simulink model "BLDC_FOC_Universal_Controller"  (R2025b)
settings: Solver=ode4  StartTime=0.0  StopTime=2  FixedStep=1e-5  RelTol=1e-3
undefined symbols (not defined in the file or in its folder): CurrentMotor_Imax, CurrentMotor_J, CurrentMotor_Kt, CurrentMotor_L, CurrentMotor_P, CurrentMotor_R, CurrentMotor_SpeedRef
libraries: fl_lib x13, nesl_utility x10, slpidlib x3, mcbeeMathTransformLib x2, eeTransforms x2, ee_lib x1
settings Model: Creator=metro  LastModifiedBy=metro

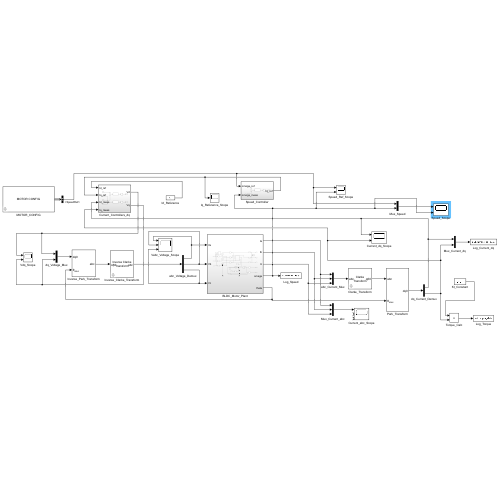
[thumbnail: Simulink's stored preview of the top-level diagram]
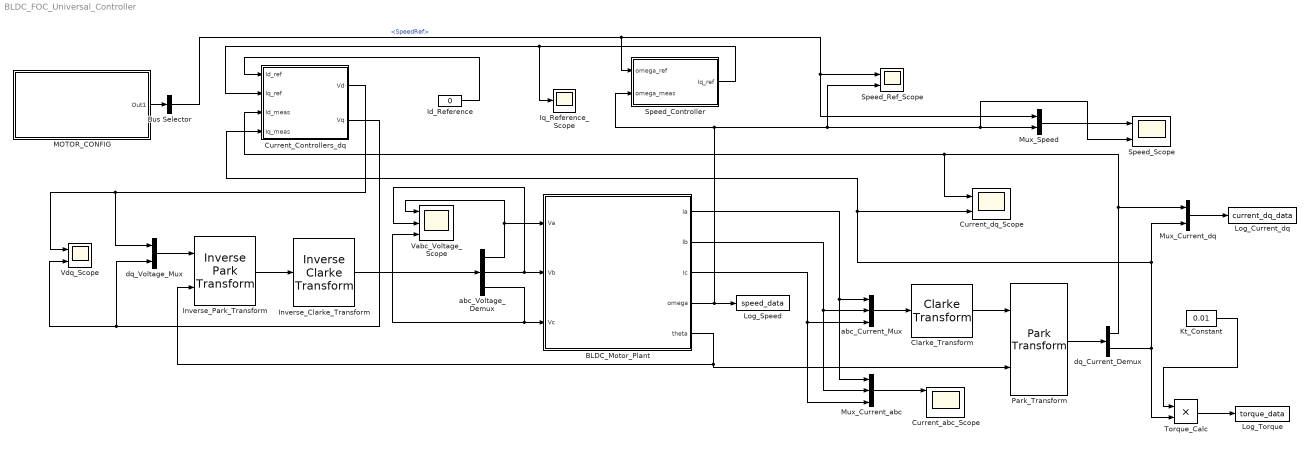
== system BLDC_FOC_Universal_Controller ==
  BLDC_Motor_Plant : Subsystem
  Bus Selector : BusSelector  OutputSignals=SpeedRef
  Clarke_Transform : mcbeeMathTransformLib/Clarke Transform  PowerInvariant=off  UseWithEmbedded=off  PhaseInput=Two inputs
      settings: LibrarySourceBlock=|
      | ee_sl_lib/Mathematical
      | Transforms/Clarke Transform
  Current_Controllers_dq : Subsystem
  Current_abc_Scope : Scope  NumInputPorts=3
      settings: ActiveDisplayYMinimum=-7.7006868638074586  ActiveDisplayYMaximum=10.228611642357857
  Current_dq_Scope : Scope  NumInputPorts=2
      settings: ActiveDisplayYMinimum=-9.97101009316468  ActiveDisplayYMaximum=4.854374604366809
  Id_Reference : Constant  Value=0
  Inverse_Clarke_Transform : mcbeeMathTransformLib/Inverse Clarke Transform  PowerInvariant=off  UseWithEmbedded=off  PhaseInput=Two inputs
      settings: LibrarySourceBlock=|
      | ee_sl_lib/Mathematical
      | Transforms/Inverse
      | Clarke Transform
  Inverse_Park_Transform : eeTransforms/Inverse Park Transform  AxisAlignment=Q-axis  PowerInvariant=off
      settings: LibrarySourceBlock=|
      | ee_sl_lib/Mathematical
      | Transforms/Inverse
      | Park Transform
  Iq_Reference_Scope : Scope
      settings: ActiveDisplayYMinimum=-2.1413567415762307  ActiveDisplayYMaximum=10.523137514468729
  Kt_Constant : Constant  Value=0.01
  Log_Current_dq : ToWorkspace  VariableName=current_dq_data  SaveFormat=Timeseries  SampleTime=-1
  Log_Speed : ToWorkspace  VariableName=speed_data  SaveFormat=Timeseries  SampleTime=-1
  Log_Torque : ToWorkspace  VariableName=torque_data  SaveFormat=Timeseries  SampleTime=-1
  MOTOR_CONFIG : Subsystem  mask{MotorType=Large Motor (2kW, 96V, 20A, 8-pole, 2000 RPM), Display_R=0.20, Display_L=0.0015, Display_Kt=0.250, Display_Imax=20.0, Display_Speed=2000}
      mask prompts: MotorType "Motor Configuration:"; Display_R "Phase Resistance (Ω):"; Display_L "Phase Inductance (H):"; Display_Kt "Torque Constant (Nm/A):"; Display_Speed "Phase Resistance (Ω):"
      mask TypeOptions MotorType: Small Motor (100W, 24V, 3A, 4-pole, 3000 RPM) | Medium Motor (500W, 48V, 10A, 6-pole, 2500 RPM) | Large Motor (2kW, 96V, 20A, 8-pole, 2000 RPM)
      mask Display: disp('MOTOR CONFIG')
  Mux_Current_abc : Mux  Inputs=3
  Mux_Current_dq : Mux  Inputs=2
  Mux_Speed : Mux  Inputs=2
  Park_Transform : eeTransforms/Park Transform  AxisAlignment=Q-axis  PowerInvariant=off
      settings: LibrarySourceBlock=|
      | ee_sl_lib/Mathematical
      | Transforms/Park Transform
  Speed_Controller : Subsystem
  Speed_Ref_Scope : Scope  NumInputPorts=2
      settings: ActiveDisplayYMinimum=-737.8438846636833  ActiveDisplayYMaximum=909.72585571077673
  Speed_Scope : Scope  NumInputPorts=2
      settings: ActiveDisplayYMinimum=-1768.9863335155014  ActiveDisplayYMaximum=1953.627322166129
  Torque_Calc : Product
  Vabc_Voltage_Scope : Scope  NumInputPorts=3
      settings: ActiveDisplayYMinimum=-17.864956119714616  ActiveDisplayYMaximum=17.127161799721005
  Vdq_Scope : Scope  NumInputPorts=2
      settings: ActiveDisplayYMinimum=-17.186680317094211  ActiveDisplayYMaximum=16.116122853847891
  abc_Current_Mux : Mux  Inputs=3
  abc_Voltage_Demux : Demux  Outputs=3
  dq_Current_Demux : Demux  Outputs=2
  dq_Voltage_Mux : Mux  Inputs=2
  wires:
  BLDC_Motor_Plant/4(omega) -> Log_Speed/1, Speed_Scope/2, Mux_Speed/2, Speed_Ref_Scope/2, Speed_Controller/2(omega_meas)
  Id_Reference/1 -> Current_Controllers_dq/1(Id_ref)
  Speed_Controller/1(Iq_ref) -> Iq_Reference_Scope/1, Current_Controllers_dq/2(Iq_ref)
  Current_Controllers_dq/1(Vd) -> Vdq_Scope/1, dq_Voltage_Mux/1
  Current_Controllers_dq/2(Vq) -> Vdq_Scope/2, dq_Voltage_Mux/2
  dq_Voltage_Mux/1 -> Inverse_Park_Transform/1
  BLDC_Motor_Plant/5(theta) -> Park_Transform/2, Inverse_Park_Transform/2
  Inverse_Park_Transform/1 -> Inverse_Clarke_Transform/1
  Inverse_Clarke_Transform/1 -> abc_Voltage_Demux/1
  abc_Voltage_Demux/1 -> Vabc_Voltage_Scope/1, BLDC_Motor_Plant/1(Va)
  abc_Voltage_Demux/2 -> BLDC_Motor_Plant/2(Vb), Vabc_Voltage_Scope/2
  abc_Voltage_Demux/3 -> Vabc_Voltage_Scope/3, BLDC_Motor_Plant/3(Vc)
  BLDC_Motor_Plant/1(Ia) -> Mux_Current_abc/1, abc_Current_Mux/1
  BLDC_Motor_Plant/2(Ib) -> Mux_Current_abc/2, abc_Current_Mux/2
  BLDC_Motor_Plant/3(Ic) -> Mux_Current_abc/3, abc_Current_Mux/3
  abc_Current_Mux/1 -> Clarke_Transform/1
  Clarke_Transform/1 -> Park_Transform/1
  Park_Transform/1 -> dq_Current_Demux/1
  Mux_Speed/1 -> Speed_Scope/1
  Mux_Current_abc/1 -> Current_abc_Scope/1
  Kt_Constant/1 -> Torque_Calc/1
  Torque_Calc/1 -> Log_Torque/1
  dq_Current_Demux/1 -> Current_Controllers_dq/3(Id_meas), Current_dq_Scope/1, Mux_Current_dq/1
  dq_Current_Demux/2 -> Mux_Current_dq/2, Current_Controllers_dq/4(Iq_meas), Current_dq_Scope/2, Torque_Calc/2
  Mux_Current_dq/1 -> Log_Current_dq/1
  MOTOR_CONFIG/1(Out1) -> Bus Selector/1
  Bus Selector/1 -> Speed_Controller/1(omega_ref), Mux_Speed/1, Speed_Ref_Scope/1  "<SpeedRef>"

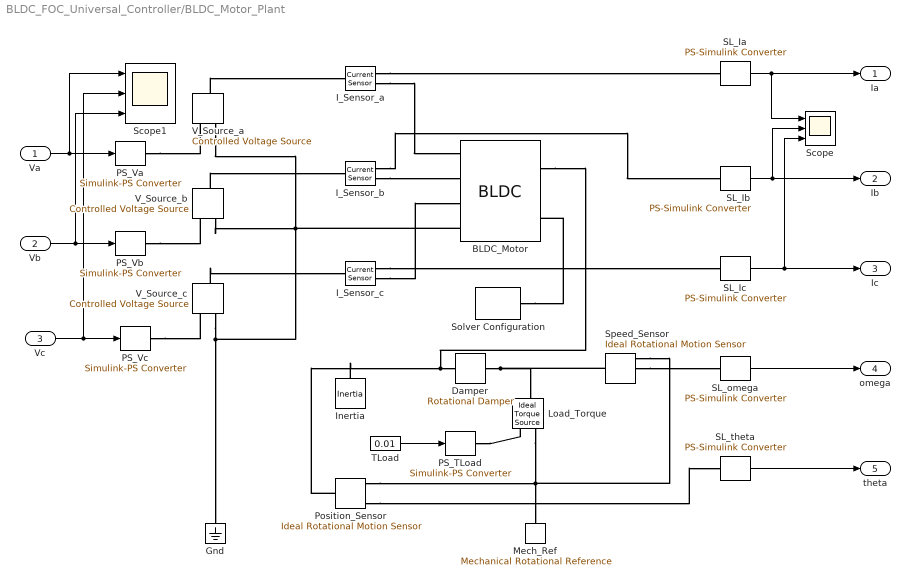
== system BLDC_FOC_Universal_Controller/BLDC_Motor_Plant ==
  Va : Inport
  Vb : Inport  Port=2
  Vc : Inport  Port=3
  BLDC_Motor : ee_lib/Electromechanical/Permanent Magnet/BLDC  port_option=ee.enum.threePhasePort.expanded  rotor_param=ee.enum.pmsm.backemf.trapezoidflux  pm_flux_linkage=CurrentMotor_Kt Wb  theta_constant=pi / 12 rad  emf_max=9.6 V  w_meas=600 rpm  DphiDtheta_tab=[0, -.1528, -.1528, .1528, .1528, 0] Wb/rad  back_emf_tab=[0, -9.6, -9.6, 9.6, 9.6, 0] V  rotor_angle_tab=[0, 7.5, 22.5, 37.5, 52.5, 60] deg  nPolePairs=CurrentMotor_P  axes_param=ee.enum.rotorangle.daxis  winding_type=ee.enum.electromech.statorconfiguration.wye  stator_param=ee.enum.statorparam.LdLqL0  machine_param=ee.enum.dqparameterization.constant  Ld=CurrentMotor_L H  Lq=CurrentMotor_L H  idVec=[-200, 0, 200] A  iqVec=[-200, 0, 200] A  LdMatrix=0.00022 * ones(3, 3) H  LqMatrix=0.00022 * ones(3, 3) H  L0=0.00016 H  Ls=0.0002 H  Lm=0 H  Ms=0.00002 H  Rs=CurrentMotor_R Ohm  zero_sequence=ee.enum.park.zerosequence.include  loss_param=ee.enum.ironloss.none  losses_oc=[0, 0, 0] W  losses_sc=[0, 0, 0] W  f_losses=60 Hz  Isc_losses=95 A  J=CurrentMotor_J kg*m^2  lam=0 N*m*s/rad  i_d_specify=off  i_d_priority=None  i_d=0 A  i_d_nominal_specify=off  i_d_nominal_value=1  i_d_nominal_unit=A  i_q_specify=off  i_q_priority=None  i_q=0 A  i_q_nominal_specify=off  i_q_nominal_value=1  i_q_nominal_unit=A  torque_specify=off  torque_priority=None  torque=0 N*m  torque_nominal_specify=off  torque_nominal_value=1  torque_nominal_unit=N*m  angular_velocity_specify=on  angular_velocity_priority=High  angular_velocity=CurrentMotor_InitialSpeed rad/s  angular_velocity_nominal_specify=off  angular_velocity_nominal_value=1  angular_velocity_nominal_unit=rpm  angular_position_specify=on  angular_position_priority=High  angular_position=0 rad  angular_position_nominal_specify=off  angular_position_nominal_value=1  angular_position_nominal_unit=deg  alpha=3.93e-3 1/K  alpha_flux=-0.001 1/K  Tmeas=298.15 K  stator_thermal_mass=100 J/K  rotor_thermal_mass=200 J/K  Rm_percent_rotor=90  Rd_percent_rotor=30  temperatureA_specify=off  temperatureA_priority=High  temperatureA=25 degC  temperatureA_nominal_specify=off  temperatureA_nominal_value=1  temperatureA_nominal_unit=degC  temperatureB_specify=off  temperatureB_priority=High  temperatureB=25 degC  temperatureB_nominal_specify=off  temperatureB_nominal_value=1  temperatureB_nominal_unit=degC  temperatureC_specify=off  temperatureC_priority=High  temperatureC=25 degC  temperatureC_nominal_specify=off  temperatureC_nominal_value=1  temperatureC_nominal_unit=degC  temperatureR_specify=off  temperatureR_priority=High  temperatureR=25 degC  temperatureR_nominal_specify=off  temperatureR_nominal_value=1  temperatureR_nominal_unit=degC
      settings: InternalSimscapePortConfiguration="{\"Bottom\":[],\"Left\":[{\"id\":\"a\",\"label\":\"a\",\"type\":\"foundation.electrical.electrical\"},{\"id\":\"b\",\"label\":\"b\",\"type\":\"foundation.electrical.electrical\"},{\"id\":\"c\",\"label\":\"c\",\"type\":\"foundation.electrical.electrical\"},{\"id\":\"n\",\"label\":\"n\",\"type\":\"foundation.electrical.electrical\"}],\"Right\":[{\"id\":\"R\",\"label\":\"R\",\"type\":\"foundation.mechanical.rotational.rotational\"},{\"id\":\"C\",\"label\":\"C\",\"type\":\"foundation.mechanical.rotational.rotational\"}],\"Top\":[]}"
  Damper : fl_lib/Mechanical/Rotational Elements/Rotational Damper  D=1e-05 N*m*s/rad  w_specify=off  w_priority=None  w=0 rad/s  w_nominal_specify=off  w_nominal_value=1  w_nominal_unit=rad/s  t_specify=off  t_priority=None  t=0 N*m  t_nominal_specify=off  t_nominal_value=1  t_nominal_unit=N*m
  Gnd : fl_lib/Electrical/Electrical Elements/Electrical Reference
  I_Sensor_a : fl_lib/Electrical/Electrical Sensors/Current Sensor
  I_Sensor_b : fl_lib/Electrical/Electrical Sensors/Current Sensor
  I_Sensor_c : fl_lib/Electrical/Electrical Sensors/Current Sensor
  Inertia : fl_lib/Mechanical/Rotational Elements/Inertia  inertia=0.0001 kg*m^2  num_ports=foundation.enum.numPorts2.one  w_specify=off  w_priority=High  w=0 rad/s  w_nominal_specify=off  w_nominal_value=1  w_nominal_unit=rad/s  t_specify=off  t_priority=None  t=0 N*m  t_nominal_specify=off  t_nominal_value=1  t_nominal_unit=N*m
  Load_Torque : fl_lib/Mechanical/Mechanical Sources/Ideal Torque Source
  Mech_Ref : fl_lib/Mechanical/Rotational Elements/Mechanical Rotational Reference
  PS_TLoad : nesl_utility/Simulink-PS Converter  PhysicalDomain=network_engine_domain  SubClassName=ps_input  LeftPortType=input  RightPortType=output  PseudoPeriodic=off  Frequencies=[]  NoiseDistribution=none  NoiseParameters=[]  Unit=1  AffineConversion=off  FilteringAndDerivatives=provide  SimscapeFilterOrder=1  InputFilterTimeConstant=0.001  UdotUserProvided=0
  PS_Va : nesl_utility/Simulink-PS Converter  PhysicalDomain=network_engine_domain  SubClassName=ps_input  LeftPortType=input  RightPortType=output  PseudoPeriodic=off  Frequencies=[]  NoiseDistribution=none  NoiseParameters=[]  Unit=1  AffineConversion=off  FilteringAndDerivatives=filter  SimscapeFilterOrder=1  InputFilterTimeConstant=0.001  UdotUserProvided=0
  PS_Vb : nesl_utility/Simulink-PS Converter  PhysicalDomain=network_engine_domain  SubClassName=ps_input  LeftPortType=input  RightPortType=output  PseudoPeriodic=off  Frequencies=[]  NoiseDistribution=none  NoiseParameters=[]  Unit=1  AffineConversion=off  FilteringAndDerivatives=filter  SimscapeFilterOrder=1  InputFilterTimeConstant=0.001  UdotUserProvided=0
  PS_Vc : nesl_utility/Simulink-PS Converter  PhysicalDomain=network_engine_domain  SubClassName=ps_input  LeftPortType=input  RightPortType=output  PseudoPeriodic=off  Frequencies=[]  NoiseDistribution=none  NoiseParameters=[]  Unit=1  AffineConversion=off  FilteringAndDerivatives=filter  SimscapeFilterOrder=1  InputFilterTimeConstant=0.001  UdotUserProvided=0
  Position_Sensor : fl_lib/Mechanical/Mechanical Sensors/Ideal Rotational Motion Sensor  reference=foundation.enum.MeasurementReference.difference  acceleration_port=false  velocity_port=true  position_port=true  wrap_angle=false  offset=0 rad
  SL_Ia : nesl_utility/PS-Simulink Converter  PhysicalDomain=network_engine_domain  SubClassName=ps_output  LeftPortType=input  RightPortType=output  PseudoPeriodic=off  Frequencies=[]  VectorFormat=inherit  Unit=inherit  AffineConversion=off
  SL_Ib : nesl_utility/PS-Simulink Converter  PhysicalDomain=network_engine_domain  SubClassName=ps_output  LeftPortType=input  RightPortType=output  PseudoPeriodic=off  Frequencies=[]  VectorFormat=inherit  Unit=inherit  AffineConversion=off
  SL_Ic : nesl_utility/PS-Simulink Converter  PhysicalDomain=network_engine_domain  SubClassName=ps_output  LeftPortType=input  RightPortType=output  PseudoPeriodic=off  Frequencies=[]  VectorFormat=inherit  Unit=inherit  AffineConversion=off
  SL_omega : nesl_utility/PS-Simulink Converter  PhysicalDomain=network_engine_domain  SubClassName=ps_output  LeftPortType=input  RightPortType=output  PseudoPeriodic=off  Frequencies=[]  VectorFormat=inherit  Unit=inherit  AffineConversion=off
  SL_theta : nesl_utility/PS-Simulink Converter  PhysicalDomain=network_engine_domain  SubClassName=ps_output  LeftPortType=input  RightPortType=output  PseudoPeriodic=off  Frequencies=[]  VectorFormat=inherit  Unit=inherit  AffineConversion=off
  Scope : Scope  NumInputPorts=3
      settings: ActiveDisplayYMinimum=-5.4784129103519961  ActiveDisplayYMaximum=2.960589649898238
  Scope1 : Scope  NumInputPorts=3
      settings: ActiveDisplayYMinimum=-35.40466722828706  ActiveDisplayYMaximum=32.32243158970072  DataLoggingVariableName=ScopeData2
  Solver Configuration : nesl_utility/Solver Configuration  PhysicalDomain=network_engine_domain  SubClassName=solver  LeftPortType=input  RightPortType=generic  Tones=[]  Harmonics=[]  SimulateNoise=off  Profile=off  UseLocalSampling=off  EnableSwitchedLinearOptims=on  FrequencyDomain=off  UseCCode=off  RelTol=0.001  AbsTol=0.001  MinStep=1e-09  ToWorkspace=off  RevertToSquareIcSolve=off  NumHomotopyIterations=100  PhasorMode=off  PhasorModeNumHarmonics=1  ConsistencySolver=NEWTON_XTOL_AFTER_FTOL  IndexReductionMethod=DerivativeReplacement  DoDC=off  ResidualTolerance=1e-09  ConsistencyTolSource=GLOBAL  ConsistencyAbsTol=0.001  ConsistencyRelTol=0.001  ConsistencyTolFactor=0.001  UseLocalSolver=off  LocalSolverChoice=NE_BACKWARD_EULER_ADVANCER  ResolveIndetEquations=on  FunctionEvalNumThread=1  LocalSolverSampleTime=0.001  DoFixedCost=off  MaxNonlinIter=3  MaxModeIter=2  ComputeImpulses=off  ImpulseIterations=2  LinearAlgebra=auto  LinearAlgebraNumThread=0  EquationFormulation=NE_TIME_EF  DelaysMemoryBudget=1024  AutomaticFiltering=on  FilteringTimeConstant=0.001  PartitionStorageMethod=AS_NEEDED  PartitionMemoryBudget=1024  PartitionMethod=ROBUST  MultibodyUseLocalSolver=off  MultibodyLocalSolverChoice=ODE1  MultibodyLocalSolverSampleTime=0.001
  Speed_Sensor : fl_lib/Mechanical/Mechanical Sensors/Ideal Rotational Motion Sensor  reference=foundation.enum.MeasurementReference.difference  acceleration_port=false  velocity_port=true  position_port=true  wrap_angle=false  offset=0 rad
  TLoad : Constant  Value=0.01
  V_Source_a : fl_lib/Electrical/Electrical Sources/Controlled Voltage Source
  V_Source_b : fl_lib/Electrical/Electrical Sources/Controlled Voltage Source
  V_Source_c : fl_lib/Electrical/Electrical Sources/Controlled Voltage Source
  Ia : Outport
  Ib : Outport  Port=2
  Ic : Outport  Port=3
  omega : Outport  Port=4
  theta : Outport  Port=5
  wires:
  Va/1 -> Scope1/1, PS_Va/1
  Vb/1 -> Scope1/3, PS_Vb/1
  Vc/1 -> Scope1/2, PS_Vc/1
  TLoad/1 -> PS_TLoad/1
  SL_Ia/1 -> Scope/1, Ia/1
  SL_Ib/1 -> Ib/1, Scope/2
  SL_Ic/1 -> Ic/1, Scope/3
  SL_omega/1 -> omega/1
  SL_theta/1 -> theta/1
  connections:
  V_Source_a/LConn1 -- I_Sensor_a/LConn1
  V_Source_b/LConn1 -- I_Sensor_b/LConn1
  V_Source_c/LConn1 -- I_Sensor_c/LConn1
  PS_Va/RConn1 -- V_Source_a/RConn1
  PS_Vb/RConn1 -- V_Source_b/RConn1
  PS_Vc/RConn1 -- V_Source_c/RConn1
  V_Source_a/RConn2 -- BLDC_Motor/LConn4 -- V_Source_b/RConn2 -- Gnd/LConn1 -- V_Source_c/RConn2
  Damper/RConn1 -- Speed_Sensor/LConn1 -- Load_Torque/LConn1 -- Position_Sensor/LConn1
  Load_Torque/RConn2 -- Position_Sensor/RConn1 -- Mech_Ref/LConn1 -- Speed_Sensor/RConn1
  PS_TLoad/RConn1 -- Load_Torque/RConn1
  I_Sensor_a/RConn1 -- SL_Ia/LConn1
  I_Sensor_b/RConn1 -- SL_Ib/LConn1
  I_Sensor_c/RConn1 -- SL_Ic/LConn1
  Speed_Sensor/RConn2 -- SL_omega/LConn1
  Position_Sensor/RConn3 -- SL_theta/LConn1
  BLDC_Motor/RConn1 -- Inertia/LConn1 -- Damper/LConn1
  Solver Configuration/RConn1 -- BLDC_Motor/RConn2
  I_Sensor_a/RConn2 -- BLDC_Motor/LConn1
  I_Sensor_b/RConn2 -- BLDC_Motor/LConn2
  I_Sensor_c/RConn2 -- BLDC_Motor/LConn3

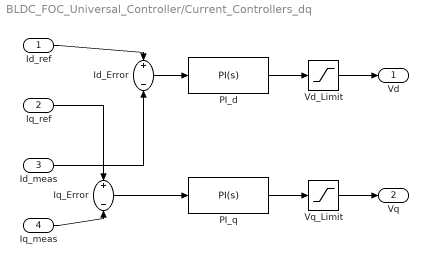
== system BLDC_FOC_Universal_Controller/Current_Controllers_dq ==
  Id_ref : Inport
  Iq_ref : Inport  Port=2
  Id_meas : Inport  Port=3
  Iq_meas : Inport  Port=4
  " Id_Error" : Sum  Inputs=+-
  " Iq_Error" : Sum  Inputs=+-
  PI_d : slpidlib/PID Controller  Controller=PI  Form=Parallel  TimeDomain=Continuous-time  UseExternalTs=off  SampleTime=-1  IntegratorMethod=Forward Euler  FilterMethod=Forward Euler  ControllerParametersSource=internal  P=5  I=50  UseKiTs=off  D=0  UseExternalDerivativeSource=off  N=100  UseFilter=on  TunerSelectOption=Transfer Function Based (PID Tuner App)  InitialConditionSource=internal  InitialConditionForIntegrator=0  InitialConditionForFilter=0  DifferentiatorICPrevScaledInput=0  ExternalReset=none  TrackingMode=off  Kt=1  LimitOutput=off  SatLimitsSource=internal  UpperSaturationLimit=inf  LowerSaturationLimit=-inf  LinearizeAsGain=on  AntiWindupMode=none  Kb=1  LimitIntegrator=off  UpperIntegratorSaturationLimit=inf  LowerIntegratorSaturationLimit=-inf  POutMin=[]  POutMax=[]  IOutMin=[]  IOutMax=[]  DOutMin=[]  DOutMax=[]  NOutMin=[]  NOutMax=[]  SumOutMin=[]  SumOutMax=[]  SaturationOutMin=[]  SaturationOutMax=[]  PParamMin=[]  PParamMax=[]  IParamMin=[]  IParamMax=[]  DParamMin=[]  DParamMax=[]  NParamMin=[]  NParamMax=[]  KbParamMin=[]  KbParamMax=[]  KtParamMin=[]  KtParamMax=[]  KbOutMin=[]  KbOutMax=[]  KtOutMin=[]  KtOutMax=[]  IntegratorOutMin=[]  IntegratorOutMax=[]  FilterOutMin=[]  FilterOutMax=[]  SumI1OutMin=[]  SumI1OutMax=[]  SumI2OutMin=[]  SumI2OutMax=[]  SumI3OutMin=[]  SumI3OutMax=[]  SumI4OutMin=[]  SumI4OutMax=[]  SumDOutMin=[]  SumDOutMax=[]  DifferentiatorOutMin=[]  DifferentiatorOutMax=[]  FilterDiffOutCoefMin=[]  FilterDiffOutCoefMax=[]  ReciprocalOutMin=[]  ReciprocalOutMax=[]  SumDenOutMin=[]  SumDenOutMax=[]  SumNumOutMin=[]  SumNumOutMax=[]  DivideOutMin=[]  DivideOutMax=[]  UdiffTsProdOutMin=[]  UdiffTsProdOutMax=[]  NTsProdOutMin=[]  NTsProdOutMax=[]  UintegralTsProdOutMin=[]  UintegralTsProdOutMax=[]  UngainTsProdOutMin=[]  UngainTsProdOutMax=[]  ClampingZeroOutDataTypeStr=Inherit: Inherit via back propagation  ClampingZeroOutMin=[]  ClampingZeroOutMax=[]  FilterDenConstantOutDataTypeStr=Inherit: Inherit via back propagation  FilterDenConstantOutMin=[]  FilterDenConstantOutMax=[]  PCopyOutDataTypeStr=Inherit: Inherit via back propagation  PCopyOutMin=[]  PCopyOutMax=[]  NCopyOutDataTypeStr=Inherit: Inherit via back propagation  NCopyOutMin=[]  NCopyOutMax=[]  IntegratorContinuousStateAttributes=''  IntegratorStateMustResolveToSignalObject=off  IntegratorRTWStateStorageClass=Auto  FilterContinuousStateAttributes=''  FilterStateMustResolveToSignalObject=off  FilterRTWStateStorageClass=Auto  ParallelPVariant=InternalParameters  IdealPVariant=Disabled  IVariant=InternalParameters  DVariant=Disabled  IntegratorVariant=Continuous  SatVariant=Disabled  AWVariant=Passthrough  PCopyVariant=Disabled  TRVariant=Disabled  FdbkBlocksVariant=Forward  IdealPFdbkVariant=Disabled  SatFdbkVariant=Disabled  DerivativeFilterVariant=Disabled  NVariant=Disabled  NCopyVariant=Disabled_SignalSpec  FilterICVariant=Disabled  IntegratorICVariant=InternalICs  ExternalResetVariant=Disabled  TRSumVariant=Passthrough  SumFdbkVariant=Disabled  SumVariant=Sum_PI  TsampFilterVariant=InternalTs  TsampNgainVariant=Passthrough  TsampIntegralVariant=Disabled_SignalSpec  ExternalSaturationOutDataTypeStr=Inherit: Same as second input  DerivativeSourceVariant=Disabled  PreIntVariant=InternalPreInt
  PI_q : slpidlib/PID Controller  Controller=PI  Form=Parallel  TimeDomain=Continuous-time  UseExternalTs=off  SampleTime=-1  IntegratorMethod=Forward Euler  FilterMethod=Forward Euler  ControllerParametersSource=internal  P=5  I=50  UseKiTs=off  D=0  UseExternalDerivativeSource=off  N=100  UseFilter=on  TunerSelectOption=Transfer Function Based (PID Tuner App)  InitialConditionSource=internal  InitialConditionForIntegrator=0  InitialConditionForFilter=0  DifferentiatorICPrevScaledInput=0  ExternalReset=none  TrackingMode=off  Kt=1  LimitOutput=off  SatLimitsSource=internal  UpperSaturationLimit=inf  LowerSaturationLimit=-inf  LinearizeAsGain=on  AntiWindupMode=none  Kb=1  LimitIntegrator=off  UpperIntegratorSaturationLimit=inf  LowerIntegratorSaturationLimit=-inf  POutMin=[]  POutMax=[]  IOutMin=[]  IOutMax=[]  DOutMin=[]  DOutMax=[]  NOutMin=[]  NOutMax=[]  SumOutMin=[]  SumOutMax=[]  SaturationOutMin=[]  SaturationOutMax=[]  PParamMin=[]  PParamMax=[]  IParamMin=[]  IParamMax=[]  DParamMin=[]  DParamMax=[]  NParamMin=[]  NParamMax=[]  KbParamMin=[]  KbParamMax=[]  KtParamMin=[]  KtParamMax=[]  KbOutMin=[]  KbOutMax=[]  KtOutMin=[]  KtOutMax=[]  IntegratorOutMin=[]  IntegratorOutMax=[]  FilterOutMin=[]  FilterOutMax=[]  SumI1OutMin=[]  SumI1OutMax=[]  SumI2OutMin=[]  SumI2OutMax=[]  SumI3OutMin=[]  SumI3OutMax=[]  SumI4OutMin=[]  SumI4OutMax=[]  SumDOutMin=[]  SumDOutMax=[]  DifferentiatorOutMin=[]  DifferentiatorOutMax=[]  FilterDiffOutCoefMin=[]  FilterDiffOutCoefMax=[]  ReciprocalOutMin=[]  ReciprocalOutMax=[]  SumDenOutMin=[]  SumDenOutMax=[]  SumNumOutMin=[]  SumNumOutMax=[]  DivideOutMin=[]  DivideOutMax=[]  UdiffTsProdOutMin=[]  UdiffTsProdOutMax=[]  NTsProdOutMin=[]  NTsProdOutMax=[]  UintegralTsProdOutMin=[]  UintegralTsProdOutMax=[]  UngainTsProdOutMin=[]  UngainTsProdOutMax=[]  ClampingZeroOutDataTypeStr=Inherit: Inherit via back propagation  ClampingZeroOutMin=[]  ClampingZeroOutMax=[]  FilterDenConstantOutDataTypeStr=Inherit: Inherit via back propagation  FilterDenConstantOutMin=[]  FilterDenConstantOutMax=[]  PCopyOutDataTypeStr=Inherit: Inherit via back propagation  PCopyOutMin=[]  PCopyOutMax=[]  NCopyOutDataTypeStr=Inherit: Inherit via back propagation  NCopyOutMin=[]  NCopyOutMax=[]  IntegratorContinuousStateAttributes=''  IntegratorStateMustResolveToSignalObject=off  IntegratorRTWStateStorageClass=Auto  FilterContinuousStateAttributes=''  FilterStateMustResolveToSignalObject=off  FilterRTWStateStorageClass=Auto  ParallelPVariant=InternalParameters  IdealPVariant=Disabled  IVariant=InternalParameters  DVariant=Disabled  IntegratorVariant=Continuous  SatVariant=Disabled  AWVariant=Passthrough  PCopyVariant=Disabled  TRVariant=Disabled  FdbkBlocksVariant=Forward  IdealPFdbkVariant=Disabled  SatFdbkVariant=Disabled  DerivativeFilterVariant=Disabled  NVariant=Disabled  NCopyVariant=Disabled_SignalSpec  FilterICVariant=Disabled  IntegratorICVariant=InternalICs  ExternalResetVariant=Disabled  TRSumVariant=Passthrough  SumFdbkVariant=Disabled  SumVariant=Sum_PI  TsampFilterVariant=InternalTs  TsampNgainVariant=Passthrough  TsampIntegralVariant=Disabled_SignalSpec  ExternalSaturationOutDataTypeStr=Inherit: Same as second input  DerivativeSourceVariant=Disabled  PreIntVariant=InternalPreInt
  Vd_Limit : Saturate  UpperLimit=13.8564  LowerLimit=-13.8564
  Vq_Limit : Saturate  UpperLimit=13.8564  LowerLimit=-13.8564
  Vd : Outport
  Vq : Outport  Port=2
  wires:
  Id_ref/1 -> " Id_Error"/1
  Id_meas/1 -> " Id_Error"/2
  " Id_Error"/1 -> PI_d/1
  PI_d/1 -> Vd_Limit/1
  Vd_Limit/1 -> Vd/1
  Iq_ref/1 -> " Iq_Error"/1
  Iq_meas/1 -> " Iq_Error"/2
  " Iq_Error"/1 -> PI_q/1
  PI_q/1 -> Vq_Limit/1
  Vq_Limit/1 -> Vq/1

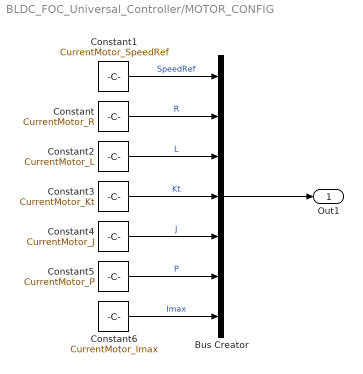
== system BLDC_FOC_Universal_Controller/MOTOR_CONFIG ==
  Bus Creator : BusCreator  Inputs=7
  Constant : Constant  Value=CurrentMotor_R
  Constant1 : Constant  Value=CurrentMotor_SpeedRef
  Constant2 : Constant  Value=CurrentMotor_L
  Constant3 : Constant  Value=CurrentMotor_Kt
  Constant4 : Constant  Value=CurrentMotor_J
  Constant5 : Constant  Value=CurrentMotor_P
  Constant6 : Constant  Value=CurrentMotor_Imax
  Out1 : Outport
  wires:
  Constant6/1 -> Bus Creator/7  "Imax"
  Constant5/1 -> Bus Creator/6  "P"
  Constant4/1 -> Bus Creator/5  "J"
  Constant3/1 -> Bus Creator/4  "Kt"
  Constant2/1 -> Bus Creator/3  "L"
  Constant/1 -> Bus Creator/2  "R"
  Constant1/1 -> Bus Creator/1  "SpeedRef"
  Bus Creator/1 -> Out1/1

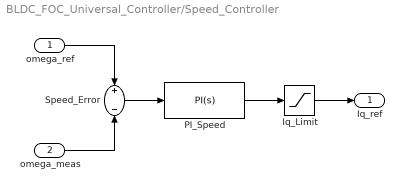
== system BLDC_FOC_Universal_Controller/Speed_Controller ==
  omega_ref : Inport
  omega_meas : Inport  Port=2
  " Speed_Error" : Sum  Inputs=+-
  Iq_Limit : Saturate  UpperLimit=3  LowerLimit=-3
  PI_Speed : slpidlib/PID Controller  Controller=PI  Form=Parallel  TimeDomain=Continuous-time  UseExternalTs=off  SampleTime=-1  IntegratorMethod=Forward Euler  FilterMethod=Forward Euler  ControllerParametersSource=internal  P=0.1  I=2  UseKiTs=off  D=0  UseExternalDerivativeSource=off  N=100  UseFilter=on  TunerSelectOption=Transfer Function Based (PID Tuner App)  InitialConditionSource=internal  InitialConditionForIntegrator=0  InitialConditionForFilter=0  DifferentiatorICPrevScaledInput=0  ExternalReset=none  TrackingMode=off  Kt=1  LimitOutput=off  SatLimitsSource=internal  UpperSaturationLimit=inf  LowerSaturationLimit=-inf  LinearizeAsGain=on  AntiWindupMode=none  Kb=1  LimitIntegrator=off  UpperIntegratorSaturationLimit=inf  LowerIntegratorSaturationLimit=-inf  POutMin=[]  POutMax=[]  IOutMin=[]  IOutMax=[]  DOutMin=[]  DOutMax=[]  NOutMin=[]  NOutMax=[]  SumOutMin=[]  SumOutMax=[]  SaturationOutMin=[]  SaturationOutMax=[]  PParamMin=[]  PParamMax=[]  IParamMin=[]  IParamMax=[]  DParamMin=[]  DParamMax=[]  NParamMin=[]  NParamMax=[]  KbParamMin=[]  KbParamMax=[]  KtParamMin=[]  KtParamMax=[]  KbOutMin=[]  KbOutMax=[]  KtOutMin=[]  KtOutMax=[]  IntegratorOutMin=[]  IntegratorOutMax=[]  FilterOutMin=[]  FilterOutMax=[]  SumI1OutMin=[]  SumI1OutMax=[]  SumI2OutMin=[]  SumI2OutMax=[]  SumI3OutMin=[]  SumI3OutMax=[]  SumI4OutMin=[]  SumI4OutMax=[]  SumDOutMin=[]  SumDOutMax=[]  DifferentiatorOutMin=[]  DifferentiatorOutMax=[]  FilterDiffOutCoefMin=[]  FilterDiffOutCoefMax=[]  ReciprocalOutMin=[]  ReciprocalOutMax=[]  SumDenOutMin=[]  SumDenOutMax=[]  SumNumOutMin=[]  SumNumOutMax=[]  DivideOutMin=[]  DivideOutMax=[]  UdiffTsProdOutMin=[]  UdiffTsProdOutMax=[]  NTsProdOutMin=[]  NTsProdOutMax=[]  UintegralTsProdOutMin=[]  UintegralTsProdOutMax=[]  UngainTsProdOutMin=[]  UngainTsProdOutMax=[]  ClampingZeroOutDataTypeStr=Inherit: Inherit via back propagation  ClampingZeroOutMin=[]  ClampingZeroOutMax=[]  FilterDenConstantOutDataTypeStr=Inherit: Inherit via back propagation  FilterDenConstantOutMin=[]  FilterDenConstantOutMax=[]  PCopyOutDataTypeStr=Inherit: Inherit via back propagation  PCopyOutMin=[]  PCopyOutMax=[]  NCopyOutDataTypeStr=Inherit: Inherit via back propagation  NCopyOutMin=[]  NCopyOutMax=[]  IntegratorContinuousStateAttributes=''  IntegratorStateMustResolveToSignalObject=off  IntegratorRTWStateStorageClass=Auto  FilterContinuousStateAttributes=''  FilterStateMustResolveToSignalObject=off  FilterRTWStateStorageClass=Auto  ParallelPVariant=InternalParameters  IdealPVariant=Disabled  IVariant=InternalParameters  DVariant=Disabled  IntegratorVariant=Continuous  SatVariant=Disabled  AWVariant=Passthrough  PCopyVariant=Disabled  TRVariant=Disabled  FdbkBlocksVariant=Forward  IdealPFdbkVariant=Disabled  SatFdbkVariant=Disabled  DerivativeFilterVariant=Disabled  NVariant=Disabled  NCopyVariant=Disabled_SignalSpec  FilterICVariant=Disabled  IntegratorICVariant=InternalICs  ExternalResetVariant=Disabled  TRSumVariant=Passthrough  SumFdbkVariant=Disabled  SumVariant=Sum_PI  TsampFilterVariant=InternalTs  TsampNgainVariant=Passthrough  TsampIntegralVariant=Disabled_SignalSpec  ExternalSaturationOutDataTypeStr=Inherit: Same as second input  DerivativeSourceVariant=Disabled  PreIntVariant=InternalPreInt
  Iq_ref : Outport
  wires:
  omega_ref/1 -> " Speed_Error"/1
  omega_meas/1 -> " Speed_Error"/2
  " Speed_Error"/1 -> PI_Speed/1
  PI_Speed/1 -> Iq_Limit/1
  Iq_Limit/1 -> Iq_ref/1
